simulink model "musule"  (R2014b)
settings: Solver=ode4  StartTime=0.0  StopTime=60  FixedStep=0.01  RelTol=1e-3
values from neighbouring files (symbols this model uses):
  n = input(prompt)    [init.m]    (also in init_consensus.m = 4; init_consensus_15.m = 15; init_mussels.m = 5; init_mussels_2.m = 5)
  sko_x = transp(sko_x)    [fishplot.m]    (also in rander.m = [0.5, 1.5, 4, 4.5, 5, 7, 8, 9.5])
  sko_y = transp(sko_y)    [fishplot.m]    (also in rander.m = [8, 3, 5, 1, 4.5, 9, 3, 6])
undefined symbols (not defined in the file or in its folder): X, Y
settings Model: Creator=Demijan  LastModifiedBy=Demijan

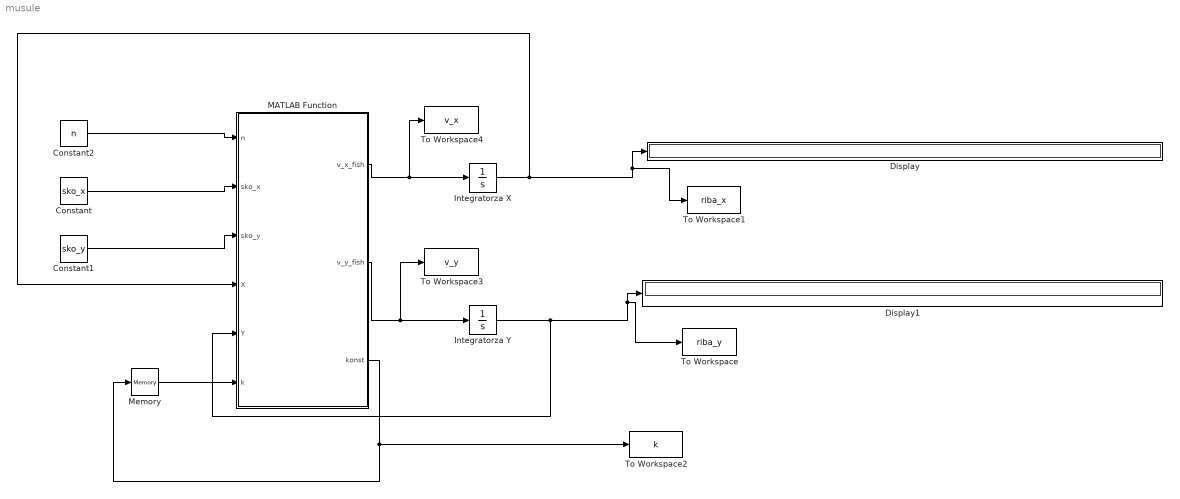
== system musule ==
  Constant : Constant  Value=sko_x
  Constant1 : Constant  Value=sko_y
  Constant2 : Constant  Value=n
  Display : Display
  Display1 : Display
  Integratorza X : Integrator  InitialCondition=X  LimitOutput=on  UpperSaturationLimit=10  LowerSaturationLimit=0
  Integratorza Y : Integrator  InitialCondition=Y  LimitOutput=on  UpperSaturationLimit=10  LowerSaturationLimit=0
  MATLAB Function : MATLAB Function  TreatAsAtomicUnit=on
  Memory : Memory  X0=[1,1,1,1,1,1,1,1]  LinearizeAsDelay=on
  To Workspace : ToWorkspace  VariableName=riba_y  SaveFormat=Structure With Time  SampleTime=-1
  To Workspace1 : ToWorkspace  VariableName=riba_x  SaveFormat=Structure With Time  SampleTime=-1
  To Workspace2 : ToWorkspace  VariableName=k  SaveFormat=Structure With Time  SampleTime=-1
  To Workspace3 : ToWorkspace  VariableName=v_y  SaveFormat=Structure With Time  SampleTime=-1
  To Workspace4 : ToWorkspace  VariableName=v_x  SaveFormat=Structure With Time  SampleTime=-1
  wires:
  MATLAB Function/1(v_x_fish) -> To Workspace4/1, Integratorza X/1
  MATLAB Function/2(v_y_fish) -> To Workspace3/1, Integratorza Y/1
  Constant2/1 -> MATLAB Function/1(n)
  Constant1/1 -> MATLAB Function/3(sko_y)
  Constant/1 -> MATLAB Function/2(sko_x)
  Integratorza Y/1 -> MATLAB Function/5(Y), Display1/1, To Workspace/1
  Integratorza X/1 -> MATLAB Function/4(X), Display/1, To Workspace1/1
  MATLAB Function/3(konst) -> Memory/1, To Workspace2/1
  Memory/1 -> MATLAB Function/6(k)

== matlab function musule/MATLAB Function ==
  data: n input; v_x_fish output; sko_x input; sko_y input; v_y_fish output; X input; Y input; k input; konst output
function [v_x_fish,v_y_fish,konst] = fcn(n,sko_x, sko_y, X, Y, k) 
        d=[0; 0; 0; 0; 0; 0; 0; 0];
        red=zeros(8,8);
        red(1,:)=[4 8 6 5 3 7 1 4];
        red(2,:)=[1 2 3 4 5 6 7 8];
        red(3,:)=[8 6 2 4 3 4 2 5];
        red(4,:)=[2 7 2 7 4 5 1 8];
        red(5,:)=[5 3 6 1 8 5 6 3];
        red(6,:)=[7 8 4 3 6 1 7 2];
        red(7,:)=[5 3 7 6 8 2 1 4];
        red(8,:)=[4 5 4 5 6 7 1 3];
        d_x=[0; 0; 0; 0; 0; 0; 0; 0];
        d_y=[0; 0; 0; 0; 0; 0; 0; 0];
        v_x_fish=[0; 0; 0; 0; 0; 0; 0; 0];
        v_y_fish=[0; 0; 0; 0; 0; 0; 0; 0];
for i=1:n;
   d_x(i)=(sko_x(red(k(i),i))-X(i));
   d_y(i)=(sko_y(red(k(i),i))-Y(i));
   d(i)=sqrt(d_x(i)^2+d_y(i)^2);
    if(d(i)<=0.01);
       k(i)=k(i)+1;
       if(k(i)>=9);
           k(i)=1;
       end
    end
   v_x_fish(i)=(d_x(i)/d(i));
   v_y_fish(i)=(d_y(i)/d(i));
end
konst=k;
end
